simulink model "sample04_speed_pd"  (R2023a)
settings: Solver=ode1  StartTime=0.0  StopTime=inf  FixedStep=0.005  RelTol=1e-3  EnableMultiTasking=on
libraries: roller485lib x3
settings Model: ExtModeTrigDuration=2  Creator=kawata  LastModifiedBy=kawata
settings SolverCC: AutoInsertRateTranBlk=on
settings DataIOCC: ReturnWorkspaceOutputs=off
settings OptimizationCC: EnhancedBackFolding=on  PassReuseOutputArgsAs=Individual arguments  ZeroExternalMemoryAtStartup=off  ZeroInternalMemoryAtStartup=off  MaxStackSize=64  OptimizeBlockOrder=speed  DifferentSizesBufferReuse=on  OptimizationCustomize=off  EfficientTunableParamExpr=on
settings DebuggingCC: ParameterTunabilityLossMsg=error
settings HardwareCC: ProdBitPerInt=16  ProdBitPerPointer=16  ProdBitPerSizeT=16  ProdBitPerPtrDiffT=16  ProdLargestAtomicFloat=None  ProdWordSize=8  ProdHWDeviceType=Atmel->AVR  UseEmbeddedCoderFeatures=off  UseSimulinkCoderFeatures=off
settings SFSimCC: MATLABDynamicMemAlloc=off
settings RTWCC: Description=Embedded Coder  SystemTargetFile=ert.tlc  HardwareBoard=Arduino Mega 2560  TemplateMakefile=ert_default_tmf  Toolchain=Arduino AVR  BuildConfiguration=Faster Runs  GPUComputeCapability=5.0
settings CodeAppCC: ForceParamTrailComments=on  IgnoreCustomStorageClasses=off  OperatorAnnotations=on  SimulinkDataObjDesc=on  SFDataObjDesc=on  InsertBlockDesc=on
settings ERTTargetCC: SupportContinuousTime=on  SupportNonInlinedSFcns=on  SupportVariableSizeSignals=on  ExtModeTransport=3  ExtModeStaticAlloc=on  ExtModeAutomaticAllocSize=off  ExtModeStaticAllocSize=2048  ExtModeMexFile=ext_xcp  ExtModeIntrfLevel=Level2 - Open

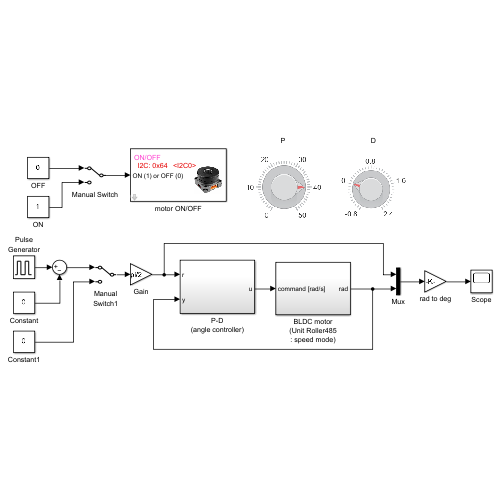
[thumbnail: Simulink's stored preview of the top-level diagram]
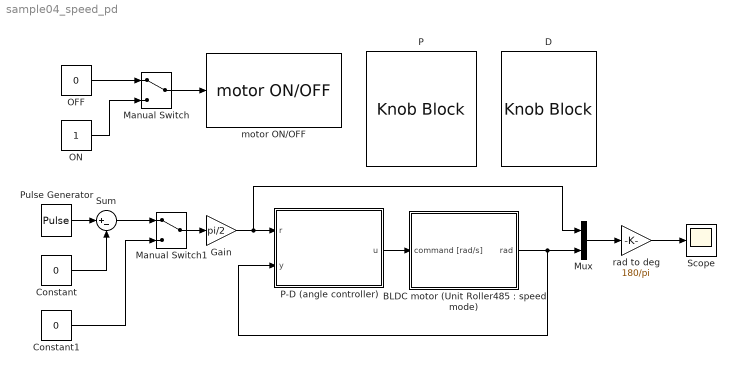
== system sample04_speed_pd ==
  "BLDC motor (Unit Roller485 : speed mode)" : Subsystem
  Constant : Constant  Value=0
  Constant1 : Constant  Value=0
  D : KnobBlock  LabelPosition=Hide  ScaleMin=-0.8  ScaleMax=2.4  TickInterval=0.8
  Gain : Gain  Gain=pi/2
  Manual Switch1 : ManualSwitch
  Manual Switch : ManualSwitch
  Mux : Mux  Inputs=2
  OFF : Constant  Value=0
  ON : Constant
  P : KnobBlock  LabelPosition=Hide  ScaleMax=50  TickInterval=10
  P-D (angle controller) : Subsystem
  Pulse Generator : DiscretePulseGenerator  PulseType=Time based  Period=4  PulseWidth=50  PhaseDelay=1
  Scope : Scope
  Sum : Sum  Inputs=|+-
  motor ON/OFF : roller485lib/motor ON//OFF  I2CAddress=0x64  I2CModule=0
      settings: SourceProductName=Roller485 Library
  rad to deg : Gain  Gain=180/pi
  wires:
  Manual Switch/1 -> motor ON/OFF/1
  OFF/1 -> Manual Switch/1
  ON/1 -> Manual Switch/2
  Constant/1 -> Sum/2
  Pulse Generator/1 -> Sum/1
  Mux/1 -> rad to deg/1
  P-D (angle controller)/1(u) -> "BLDC motor (Unit Roller485 : speed mode)"/1(command [rad/s])
  Gain/1 -> P-D (angle controller)/1(r), Mux/1
  "BLDC motor (Unit Roller485 : speed mode)"/1(rad) -> P-D (angle controller)/2(y), Mux/2
  rad to deg/1 -> Scope/1
  Manual Switch1/1 -> Gain/1
  Sum/1 -> Manual Switch1/1
  Constant1/1 -> Manual Switch1/2

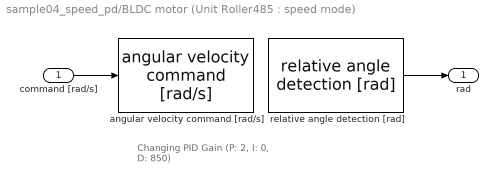
== system sample04_speed_pd/BLDC motor (Unit Roller485 : speed mode) ==
  note: Changing PID Gain
      | (P: 2, I: 0, D: 850)
  command [rad/s] : Inport
  angular velocity command [rad/s] : roller485lib/I2C Write/angular velocity command [rad//s]  I2CAddress=0x64  I2CModule=0  speed_P=2  speed_I=0  speed_D=850  set_time1=0  set_time2=0
      settings: SourceProductName=Roller485 Library
  relative angle detection [rad] : roller485lib/I2C Read/relative angle detection [rad]  I2CAddress=0x64  I2CModule=0  sample_time=-1  set_time=0
      settings: SourceProductName=Roller485 Library
  rad : Outport
  wires:
  command [rad/s]/1 -> angular velocity command [rad/s]/1
  relative angle detection [rad]/1 -> rad/1

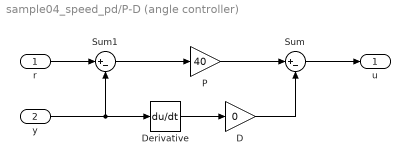
== system sample04_speed_pd/P-D (angle controller) ==
  r : Inport
  y : Inport  Port=2
  D : Gain  Gain=0
  Derivative : Derivative
  P : Gain  Gain=40
  Sum : Sum  Inputs=|+-
  Sum1 : Sum  Inputs=|+-
  u : Outport
  wires:
  Sum/1 -> u/1
  P/1 -> Sum/1
  Derivative/1 -> D/1
  r/1 -> Sum1/1
  Sum1/1 -> P/1
  y/1 -> Sum1/2, Derivative/1
  D/1 -> Sum/2
